simulink model "Vending_1"  (R2019a)
settings: Solver=VariableStepAuto  StartTime=0.0  StopTime=100  RelTol=1e-3
settings Model: EnablePacing=on  PacingRate=1.600000  Creator=kedar  LastModifiedBy=kejo5874

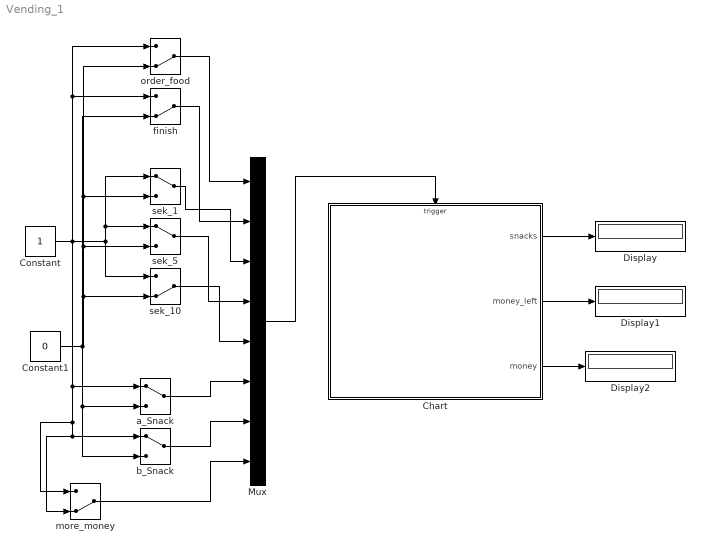
== system Vending_1 ==
  Chart : Stateflow chart  BlockKeywords=__PRM__SERIALIZED__DATA__:Stateflow Chart,Stateflow Diagram  TreatAsAtomicUnit=on
  Constant : Constant
  Constant1 : Constant  Value=0
  Display : Display
  Display1 : Display
  Display2 : Display
  Mux : Mux  Inputs=8
  a_Snack : ManualSwitch
  b_Snack : ManualSwitch
  finish : ManualSwitch  CurrentSetting=0
  more_money : ManualSwitch  CurrentSetting=0
  "order_food " : ManualSwitch  CurrentSetting=0
  sek_1 : ManualSwitch
  sek_10 : ManualSwitch  CurrentSetting=0
  sek_5 : ManualSwitch
  wires:
  Constant/1 -> more_money/1, more_money/2, b_Snack/1, a_Snack/1, finish/1, "order_food "/1, sek_5/1, sek_1/1, sek_10/1
  Constant1/1 -> b_Snack/2, a_Snack/2, finish/2, "order_food "/2, sek_1/2, sek_5/2, sek_10/2
  Mux/1 -> Chart/Trigger
  sek_1/1 -> Mux/3
  sek_5/1 -> Mux/4
  sek_10/1 -> Mux/5
  Chart/1(snacks) -> Display/1
  a_Snack/1 -> Mux/6
  b_Snack/1 -> Mux/7
  finish/1 -> Mux/2
  "order_food "/1 -> Mux/1
  more_money/1 -> Mux/8
  Chart/2(money_left) -> Display1/1
  Chart/3(money) -> Display2/1

== stateflow chart Vending_1/Chart ==
  settings: executeAtInitialization=1
  state VendingMachine
    en: money = 0;
    state MoneyCollector
      on sek_1: money = money + 1;
      on sek_5: money = money + 5;
      on sek_10: money = money + 10;
    state SnackVendor
      on a_Snack: Snack_A()
      on b_Snack: Snack_B()
    state Finish
      on finish: money_left = money
      money = 0;
    (default) -> MoneyCollector
    MoneyCollector -> SnackVendor : order_food
    SnackVendor -> MoneyCollector [order 1] : more_money
    SnackVendor -> Finish [order 2] : finish
  (default) -> VendingMachine
  data: snacks output double; money_left output; money output
  events: sek_1 input EITHER_EDGE_EVENT; sek_5 input EITHER_EDGE_EVENT; sek_10 input EITHER_EDGE_EVENT; finish input EITHER_EDGE_EVENT; more_money input EITHER_EDGE_EVENT; order_food input RISING_EDGE_EVENT; a_Snack input RISING_EDGE_EVENT; b_Snack input RISING_EDGE_EVENT
  function Snack_A:
    | 
    | function Snack_A
    | Snack_A_cost = 6;
    | if money>=6
    |     money = money - Snack_A_cost;
    |     snacks = 1;
    | else
    |     snacks = 0;
    | end
  function Snack_B:
    | 
    | function Snack_B
    | Snack_B_cost = 8;
    | if money>=8
    |     money = money - Snack_B_cost;
    |     snacks = 1;
    | else
    |     snacks = 0;
    | end
